simulink model "RaviDFG"  (R2023a)
settings: Solver=ode5  StartTime=0.0  StopTime=15  FixedStep=50e-9  MaxStep=1e-2  MinStep=1e-3  RelTol=1e-3  AbsTol=1e-3
undefined symbols (not defined in the file): d_base, d_Beta, d_bl, d_Cdc, d_Cf, d_ctg, d_GSC_IL1_iv, d_GSC_IL1_ki, d_GSC_IL1_kp, d_GSC_IL2_iv, d_GSC_IL2_ki, d_GSC_IL2_kp, d_GSC_OL1_iv, d_GSC_OL1_ki, d_GSC_OL1_kp, d_GSC_OL2_iv, d_GSC_OL2_ki, d_GSC_OL2_kp, d_Hg, d_Ht, d_igd, d_igq, d_iid, d_iiq, d_isd, d_isq, d_Kmrr, d_kopt, d_ktg, d_Lg, d_Li, d_Lm, d_Ls_d, d_MSC_IL1_iv, d_MSC_IL1_ki, d_MSC_IL1_kp, d_MSC_IL2_iv, d_MSC_IL2_ki, d_MSC_IL2_kp, d_MSC_OL1_iv, d_MSC_OL1_ki, d_MSC_OL1_kp, d_MSC_OL2_iv, d_MSC_OL2_ki, d_MSC_OL2_kp, d_Qs, d_R1, d_R2, d_Rc, d_Rg, d_Ri, d_Tr, d_Ts, d_vcd, d_vcq, d_VDC, d_vw, d_welb, d_wg, d_ws ... (+7)
libraries: eeGeneralControl x2, rtlab x2
settings Model: Creator=rpat227  LastModifiedBy=rufar
settings SolverCC: AlgebraicLoopSolver=TrustRegion
settings DebuggingCC: UnconnectedInputMsg=warning  UnconnectedOutputMsg=warning  UnconnectedLineMsg=warning
settings ModelReferenceCC: EnableRefExpFcnMdlSchedulingChecks=on

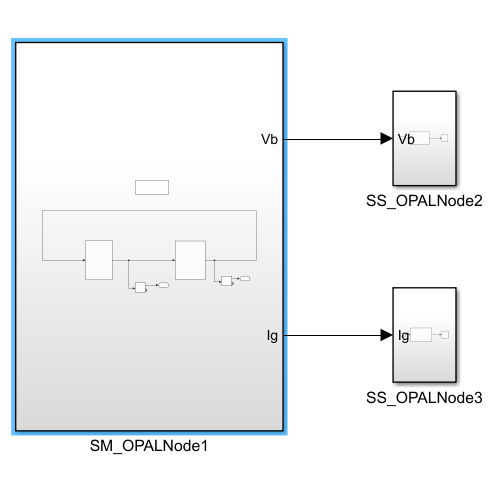
[thumbnail: Simulink's stored preview of the top-level diagram]
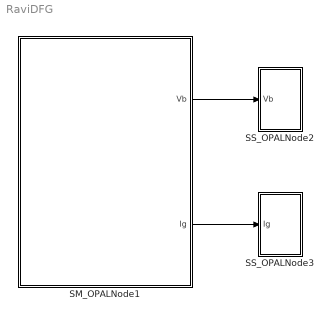
== system RaviDFG ==
  SM_OPALNode1 : Subsystem
  SS_OPALNode2 : Subsystem
  SS_OPALNode3 : Subsystem
  wires:
  SM_OPALNode1/1(Vb) -> SS_OPALNode2/1(Vb)
  SM_OPALNode1/2(Ig) -> SS_OPALNode3/1(Ig)

== system RaviDFG/SM_OPALNode1 ==
  Complex to Real-Imag : ComplexToRealImag
  Complex to Real-Imag1 : ComplexToRealImag
  DFIG : Subsystem
  Measurement : Subsystem
  Network : Subsystem
  Vb : Outport
  Ig : Outport  Port=2
  wires:
  DFIG/1(Ig) -> Complex to Real-Imag/1, Network/1(Ig)
  Network/1(Vb) -> Complex to Real-Imag1/1, DFIG/1(Vb)
  Complex to Real-Imag/1 -> Ig/1
  Complex to Real-Imag1/1 -> Vb/1

== system RaviDFG/SS_OPALNode2 ==
  Vb : Inport
  OpComm1 : rtlab/OpComm  nbport=1  groupe_acq=1  subsys_rate=0  st=0  Synchronization=on  Interpolation=on  Threshold=1.0  Missed_Data=off  Sim_Time=off  Samples=off  dynSigOut=off  from_console=0  warning_done=off  writeOpCommFile=off  Offset=off
      settings: SourceProductName=RT-LAB
  Vb_Scope : Scope
  wires:
  OpComm1/1 -> Vb_Scope/1
  Vb/1 -> OpComm1/1

== system RaviDFG/SS_OPALNode3 ==
  Ig : Inport
  Ig_Scope : Scope
  OpComm : rtlab/OpComm  nbport=1  groupe_acq=1  subsys_rate=0  st=0  Synchronization=on  Interpolation=on  Threshold=1.0  Missed_Data=off  Sim_Time=off  Samples=off  dynSigOut=off  from_console=0  warning_done=off  writeOpCommFile=off  Offset=off
      settings: SourceProductName=RT-LAB
  wires:
  OpComm/1 -> Ig_Scope/1
  Ig/1 -> OpComm/1

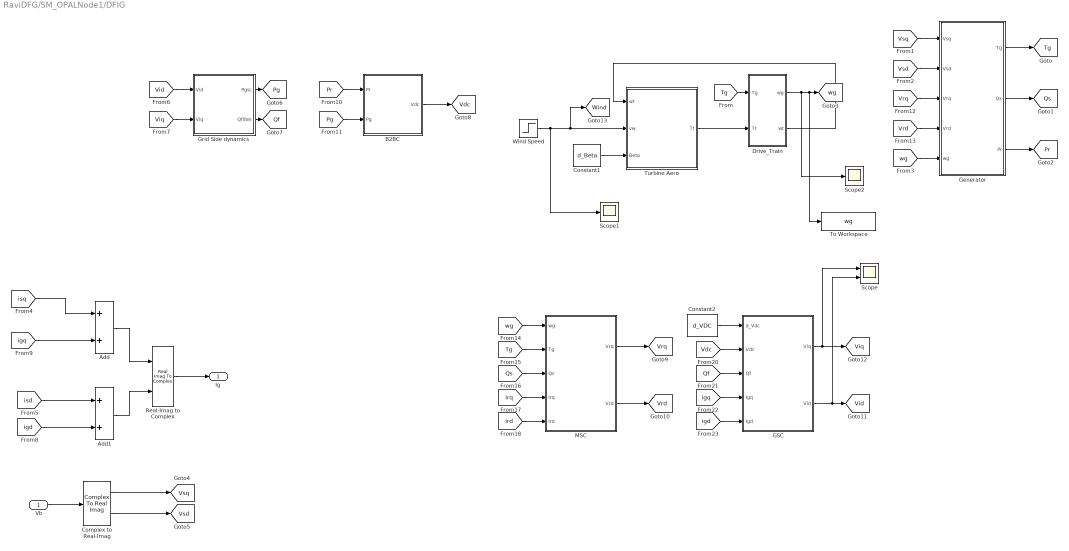
== system RaviDFG/SM_OPALNode1/DFIG ==
  Vb : Inport
  Add : Sum
  Add1 : Sum
  B2BC : Subsystem
  Complex to Real-Imag : ComplexToRealImag
  Constant1 : Constant  Value=d_Beta
  Constant2 : Constant  Value=d_VDC
  Drive_Train : Subsystem
  GSC : Subsystem
  Generator : Subsystem
  Grid Side dynamics : Subsystem
  MSC : Subsystem
  Real-Imag to Complex : RealImagToComplex
  Scope : Scope  NumInputPorts=2
  Scope1 : Scope
  Scope2 : Scope
  To Workspace : ToWorkspace  VariableName=wg  SaveFormat=Structure With Time  SampleTime=-1
  Turbine Aero : Subsystem
  Wind Speed : Step  Time=5  Before=d_vw  After=d_vw  SampleTime=0
  Ig : Outport
  tag scope: Pg=global, Pr=global, Qf=global, Qs=global, Tg=global, Vdc=global, Vid=global, Viq=global, Vrd=global, Vrq=global, Vsd=global, Vsq=global, Wind=global, wg=global
  wires:
  MSC/1(Vrq) -> [Vrq]
  [Pg] -> B2BC/2(Pg)
  [Viq] -> Grid Side dynamics/2(Viq)
  B2BC/1(Vdc) -> [Vdc]
  [Pr] -> B2BC/1(Pr)
  GSC/1(Viq) -> Scope/1, [Viq]
  Turbine Aero/1(Tt) -> Drive_Train/2(Tt)
  [irq] -> MSC/4(Irq)
  Wind Speed/1 -> Scope1/1, Turbine Aero/2(vw), [Wind]
  [Qs] -> MSC/3(Qs)
  [wg] -> MSC/1("wg ")
  Generator/3(Pr) -> [Pr]
  Drive_Train/1(wg) -> Scope2/1, To Workspace/1, [wg]
  [Qf] -> GSC/3(Qf)
  [Tg] -> MSC/2(Tg)
  Constant1/1 -> Turbine Aero/3(Beta)
  Grid Side dynamics/2(Qfilter) -> [Qf]
  [Tg] -> Drive_Train/1(Tg)
  [Vrq] -> Generator/3(Vrq)
  [Vrd] -> Generator/4(Vrd)
  [Vdc] -> GSC/2(Vdc)
  [igd] -> GSC/5(Igd)
  [Vid] -> Grid Side dynamics/1(Vid)
  Generator/2(Qs) -> [Qs]
  Generator/1(Tg) -> [Tg]
  [Vsd] -> Generator/2(Vsd)
  Grid Side dynamics/1(Pgsc) -> [Pg]
  [Vsq] -> Generator/1(Vsq)
  Drive_Train/2(wt) -> Turbine Aero/1(wt)
  [igq] -> GSC/4(Igq)
  MSC/2(Vrd) -> [Vrd]
  Constant2/1 -> GSC/1("d_Vdc ")
  GSC/2(Vid) -> Scope/2, [Vid]
  [wg] -> Generator/5(wg)
  [ird] -> MSC/5(Ird)
  [igd] -> Add1/2
  Add1/1 -> Real-Imag to Complex/2
  [igq] -> Add/2
  Add/1 -> Real-Imag to Complex/1
  [isd] -> Add1/1
  [isq] -> Add/1
  Real-Imag to Complex/1 -> Ig/1
  Vb/1 -> Complex to Real-Imag/1
  Complex to Real-Imag/2 -> [Vsd]
  Complex to Real-Imag/1 -> [Vsq]

== system RaviDFG/SM_OPALNode1/Measurement ==
  Scope{,1..7} (8 alike) : Scope
  To Workspace : ToWorkspace  VariableName=P  SaveFormat=Structure With Time  SampleTime=-1
  wires:
  [P] -> To Workspace/1, Scope/1
  [Vinf] -> Scope7/1
  [Bus] -> Scope6/1
  [Wind] -> Scope5/1
  [Vdc] -> Scope4/1
  [Qs] -> Scope3/1
  [Pr] -> Scope2/1
  [Ps] -> Scope1/1

== system RaviDFG/SM_OPALNode1/Network ==
  Ig : Inport
  Add2 : Sum
  Complex to Magnitude-Angle : ComplexToMagnitudeAngle
  Constant : Constant  Value=vinf
  Display : Display
  Display1 : Display
  Display2 : Display
  Gain : Gain  Gain=Znet
  Vb : Outport
  tag scope: Bus=global, Theta=global, Vinf=global
  wires:
  Gain/1 -> Add2/1
  Add2/1 -> Display1/1, Vb/1, Complex to Magnitude-Angle/1
  Complex to Magnitude-Angle/2 -> [Theta]
  Complex to Magnitude-Angle/1 -> Display2/1, [Bus]
  Ig/1 -> Display/1, Gain/1
  Constant/1 -> Add2/2, [Vinf]

== system RaviDFG/SM_OPALNode1/DFIG/B2BC ==
  Pr : Inport
  Pg : Inport  Port=2
  Add : Sum  Inputs=+-
  Divide : Product  Inputs=*/
  Gain : Gain  Gain=d_Cdc
  Integrator : Integrator  InitialCondition=d_VDC
  Scope : Scope
  Vdc : Outport
  wires:
  Pr/1 -> Add/1
  Pg/1 -> Add/2
  Add/1 -> Gain/1
  Gain/1 -> Divide/1
  Divide/1 -> Integrator/1
  Integrator/1 -> Divide/2, Scope/1, Vdc/1

== system RaviDFG/SM_OPALNode1/DFIG/Drive_Train ==
  Tg : Inport
  Tt : Inport  Port=2
  Add : Sum  Inputs=-+
  Add1 : Sum  Inputs=+-
  Add2 : Sum  Inputs=-+
  Add3 : Sum
  Gain : Gain  Gain=1./(2*d_Hg)
  Gain1 : Gain  Gain=1./(2*d_Ht)
  Gain2 : Gain  Gain=d_welb
  Gain3 : Gain  Gain=d_ktg
  Gain4 : Gain  Gain=d_ctg
  d_Ts : Integrator  InitialCondition=d_Ts
  d_wg : Integrator  InitialCondition=d_wg
  d_wt : Integrator  InitialCondition=d_wt
  wg : Outport
  wt : Outport  Port=2
  wires:
  Tg/1 -> Add/1
  Tt/1 -> Add1/1
  Add/1 -> Gain/1
  Add1/1 -> Gain1/1
  Gain/1 -> d_wg/1
  Gain1/1 -> d_wt/1
  d_wg/1 -> wg/1, Add2/1
  d_wt/1 -> Add2/2, wt/1
  Add2/1 -> Gain2/1
  Gain2/1 -> Gain4/1, Gain3/1
  Gain3/1 -> d_Ts/1
  d_Ts/1 -> Add3/1
  Gain4/1 -> Add3/2
  Add3/1 -> Add/2, Add1/2

== system RaviDFG/SM_OPALNode1/DFIG/GSC ==
  "d_Vdc " : Inport
  Vdc : Inport  Port=2
  Qf : Inport  Port=3
  Igq : Inport  Port=4
  Igd : Inport  Port=5
  Add{,1..3} (4 alike) : Sum  Inputs=+-
  Constant : Constant  Value=0
  GSC_IL_1 : Subsystem
  GSC_IL_2 : Subsystem
  GSC_OL_1 : Subsystem
  GSC_OL_2 : Subsystem
  Subsystem : Subsystem
  Subsystem1 : Subsystem
  Viq : Outport
  Vid : Outport  Port=2
  wires:
  "d_Vdc "/1 -> Add/1
  Vdc/1 -> Add/2
  Add/1 -> GSC_OL_1/1(In1)
  GSC_OL_1/1(Out1) -> Add1/1
  Add1/1 -> GSC_IL_1/1(In1)
  Add2/1 -> GSC_OL_2/1(In1)
  GSC_OL_2/1(Out1) -> Add3/1
  Add3/1 -> GSC_IL_2/1(In1)
  Constant/1 -> Add2/1
  Qf/1 -> Add2/2
  Subsystem/1(Igq') -> Add1/2
  Subsystem/2(Igd') -> Add3/2
  Igq/1 -> Subsystem/1(Igq)
  Igd/1 -> Subsystem/2(Igd)
  GSC_IL_1/1(Out1) -> Subsystem1/1(Viq')
  GSC_IL_2/1(Out1) -> Subsystem1/2(Vid')
  Subsystem1/1(Viq) -> Viq/1
  Subsystem1/2(Vid) -> Vid/1

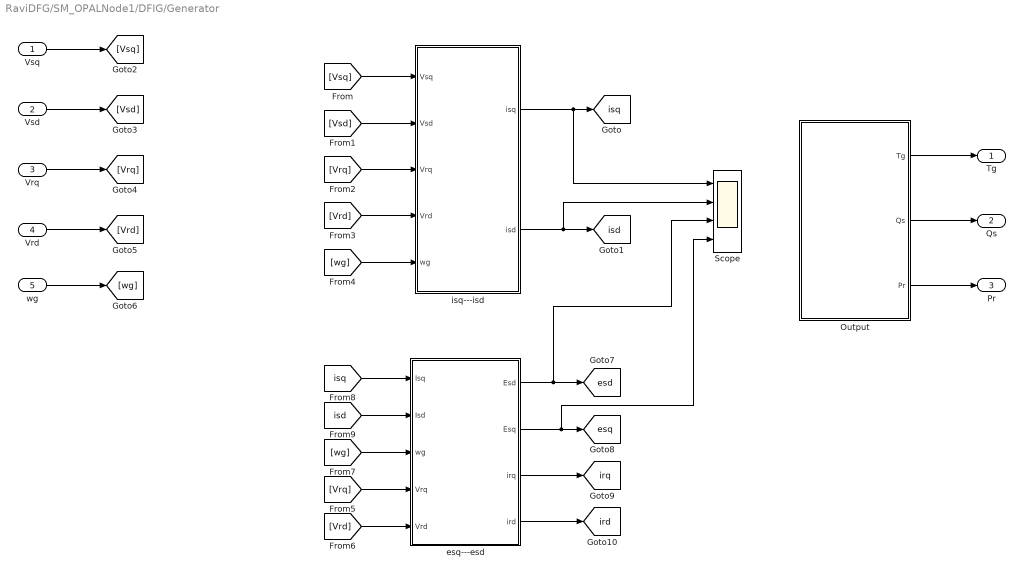
== system RaviDFG/SM_OPALNode1/DFIG/Generator ==
  Vsq : Inport
  Vsd : Inport  Port=2
  Vrq : Inport  Port=3
  Vrd : Inport  Port=4
  wg : Inport  Port=5
  Output : Subsystem
  Scope : Scope  NumInputPorts=4
  esq---esd : Subsystem
  isq---isd : Subsystem
  Tg : Outport
  Qs : Outport  Port=2
  Pr : Outport  Port=3
  tag scope: esd=global, esq=global, ird=global, irq=global, isd=global, isq=global
  wires:
  [Vsq] -> isq---isd/1(Vsq)
  [Vsd] -> isq---isd/2(Vsd)
  [Vrq] -> isq---isd/3(Vrq)
  [Vrd] -> isq---isd/4(Vrd)
  [wg] -> isq---isd/5(wg)
  isq---isd/1(isq) -> Scope/1, [isq]
  isq---isd/2(isd) -> Scope/2, [isd]
  Vsq/1 -> [Vsq]
  Vsd/1 -> [Vsd]
  Vrq/1 -> [Vrq]
  Vrd/1 -> [Vrd]
  wg/1 -> [wg]
  [Vrq] -> esq---esd/4(Vrq)
  [Vrd] -> esq---esd/5(Vrd)
  [wg] -> esq---esd/3(wg)
  [isq] -> esq---esd/1(Isq)
  [isd] -> esq---esd/2(Isd)
  esq---esd/2(Esq) -> Scope/4, [esq]
  esq---esd/3(irq) -> [irq]
  esq---esd/4(ird) -> [ird]
  Output/1(Tg) -> Tg/1
  Output/2(Qs) -> Qs/1
  Output/3(Pr) -> Pr/1
  esq---esd/1(Esd) -> Scope/3, [esd]

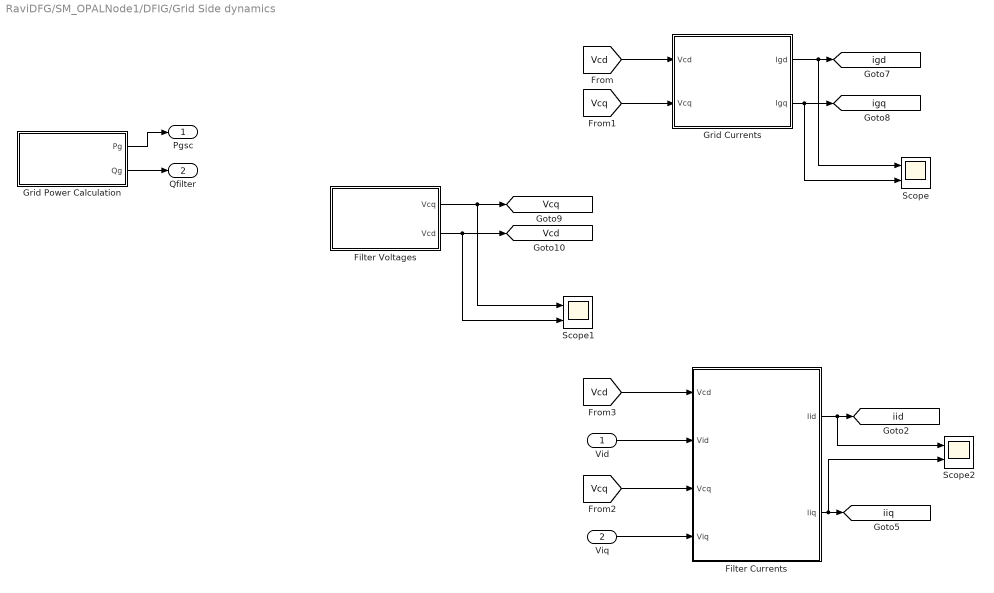
== system RaviDFG/SM_OPALNode1/DFIG/Grid Side dynamics ==
  Vid : Inport
  Viq : Inport  Port=2
  Filter Currents : Subsystem
  Filter Voltages : Subsystem
  Grid Currents : Subsystem
  Grid Power Calculation : Subsystem
  Scope : Scope  NumInputPorts=2
  Scope1 : Scope  NumInputPorts=2
  Scope2 : Scope  NumInputPorts=2
  Pgsc : Outport
  Qfilter : Outport  Port=2
  tag scope: Vcd=global, Vcq=global, igd=global, igq=global, iid=global, iiq=global
  wires:
  Grid Currents/1(Igd) -> Scope/1, [igd]
  Filter Voltages/2(Vcd) -> Scope1/2, [Vcd]
  Viq/1 -> Filter Currents/4(Viq)
  Vid/1 -> Filter Currents/2(Vid)
  [Vcd] -> Filter Currents/1(Vcd)
  [Vcq] -> Filter Currents/3(Vcq)
  Filter Voltages/1(Vcq) -> Scope1/1, [Vcq]
  [Vcq] -> Grid Currents/2(Vcq)
  Filter Currents/1(Iid) -> Scope2/1, [iid]
  Filter Currents/2(Iiq) -> Scope2/2, [iiq]
  [Vcd] -> Grid Currents/1(Vcd)
  Grid Power Calculation/1(Pg) -> Pgsc/1
  Grid Power Calculation/2(Qg) -> Qfilter/1
  Grid Currents/2(Igq) -> Scope/2, [igq]

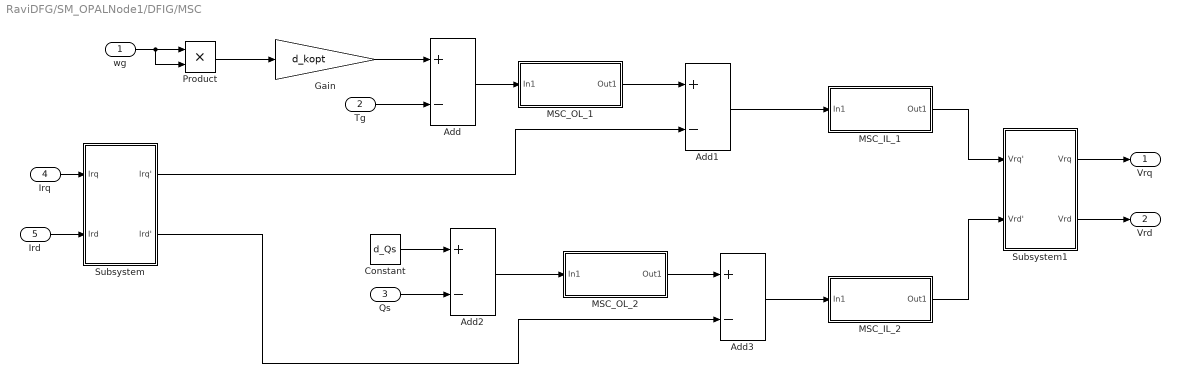
== system RaviDFG/SM_OPALNode1/DFIG/MSC ==
  "wg " : Inport
  Tg : Inport  Port=2
  Qs : Inport  Port=3
  Irq : Inport  Port=4
  Ird : Inport  Port=5
  Add{,1..3} (4 alike) : Sum  Inputs=+-
  Constant : Constant  Value=d_Qs
  Gain : Gain  Gain=d_kopt
  MSC_IL_1 : Subsystem
  MSC_IL_2 : Subsystem
  MSC_OL_1 : Subsystem
  MSC_OL_2 : Subsystem
  Product : Product
  Subsystem : Subsystem
  Subsystem1 : Subsystem
  Vrq : Outport
  Vrd : Outport  Port=2
  wires:
  "wg "/1 -> Product/2, Product/1
  Product/1 -> Gain/1
  Gain/1 -> Add/1
  Tg/1 -> Add/2
  Add/1 -> MSC_OL_1/1(In1)
  MSC_OL_1/1(Out1) -> Add1/1
  Add1/1 -> MSC_IL_1/1(In1)
  Add2/1 -> MSC_OL_2/1(In1)
  MSC_OL_2/1(Out1) -> Add3/1
  Add3/1 -> MSC_IL_2/1(In1)
  Constant/1 -> Add2/1
  Qs/1 -> Add2/2
  Subsystem/1(Irq') -> Add1/2
  Subsystem/2(Ird') -> Add3/2
  Irq/1 -> Subsystem/1(Irq)
  Ird/1 -> Subsystem/2(Ird)
  MSC_IL_1/1(Out1) -> Subsystem1/1(Vrq')
  MSC_IL_2/1(Out1) -> Subsystem1/2(Vrd')
  Subsystem1/1(Vrq) -> Vrq/1
  Subsystem1/2(Vrd) -> Vrd/1

== system RaviDFG/SM_OPALNode1/DFIG/Turbine Aero ==
  wt : Inport
  vw : Inport  Port=2
  Beta : Inport  Port=3
  Constant : Constant  Value=0.5*rho*pi*d_bl^2
  Constant4 : Constant  Value=3
  "Cp Calculation " : Subsystem
  Divide : Product  Inputs=*/
  Divide1 : Product  Inputs=*/
  Gain : Gain  Gain=d_wtrated*d_bl
  Gain1 : Gain  Gain=1/(d_base*10^6)
  Power : Math  Operator=pow
  Product : Product  Inputs=3
  Tt : Outport
  wires:
  Divide/1 -> "Cp Calculation "/1(Lambda)
  Product/1 -> Gain1/1
  Gain/1 -> Divide/1
  Power/1 -> Product/3
  vw/1 -> Power/1, Divide/2
  Constant4/1 -> Power/2
  "Cp Calculation "/1(Cp) -> Product/2
  Divide1/1 -> Tt/1
  wt/1 -> Divide1/2, Gain/1
  Beta/1 -> "Cp Calculation "/2(Beta)
  Gain1/1 -> Divide1/1
  Constant/1 -> Product/1

== system RaviDFG/SM_OPALNode1/DFIG/GSC/GSC_IL_1 ==
  In1 : Inport
  Gain : Gain  Gain=d_GSC_IL1_ki
  Gain1 : Gain  Gain=d_GSC_IL1_kp
  Integrator : Integrator  InitialCondition=d_GSC_IL1_iv
  Sum : Sum  Inputs=|++
  Out1 : Outport
  wires:
  Gain/1 -> Integrator/1
  Integrator/1 -> Sum/1
  Gain1/1 -> Sum/2
  Sum/1 -> Out1/1
  In1/1 -> Gain1/1, Gain/1

== system RaviDFG/SM_OPALNode1/DFIG/GSC/GSC_IL_2 ==
  In1 : Inport
  Gain : Gain  Gain=d_GSC_IL2_ki
  Gain1 : Gain  Gain=d_GSC_IL2_kp
  Integrator : Integrator  InitialCondition=d_GSC_IL2_iv
  Sum : Sum  Inputs=|++
  Out1 : Outport
  wires:
  Gain/1 -> Integrator/1
  Integrator/1 -> Sum/1
  Gain1/1 -> Sum/2
  Sum/1 -> Out1/1
  In1/1 -> Gain1/1, Gain/1

== system RaviDFG/SM_OPALNode1/DFIG/GSC/GSC_OL_1 ==
  In1 : Inport
  Gain : Gain  Gain=d_GSC_OL1_ki
  Gain1 : Gain  Gain=d_GSC_OL1_kp
  Integrator : Integrator  InitialCondition=d_GSC_OL1_iv
  Sum : Sum  Inputs=|++
  Out1 : Outport
  wires:
  Gain/1 -> Integrator/1
  Integrator/1 -> Sum/1
  Gain1/1 -> Sum/2
  Sum/1 -> Out1/1
  In1/1 -> Gain1/1, Gain/1

== system RaviDFG/SM_OPALNode1/DFIG/GSC/GSC_OL_2 ==
  In1 : Inport
  Gain : Gain  Gain=d_GSC_OL2_ki
  Gain1 : Gain  Gain=d_GSC_OL2_kp
  Integrator : Integrator  InitialCondition=d_GSC_OL2_iv
  Sum : Sum  Inputs=|++
  Out1 : Outport
  wires:
  Gain/1 -> Integrator/1
  Integrator/1 -> Sum/1
  Gain1/1 -> Sum/2
  Sum/1 -> Out1/1
  In1/1 -> Gain1/1, Gain/1

== system RaviDFG/SM_OPALNode1/DFIG/GSC/Subsystem ==
  Igq : Inport
  Igd : Inport  Port=2
  Complex to Real-Imag : ComplexToRealImag
  Gain : Gain  Gain=-j
  Math Function : Math
  Product : Product
  Real-Imag to Complex : RealImagToComplex
  Igq' : Outport
  Igd' : Outport  Port=2
  wires:
  Igd/1 -> Real-Imag to Complex/2
  Real-Imag to Complex/1 -> Product/1
  Gain/1 -> Math Function/1
  Complex to Real-Imag/2 -> Igd'/1
  Product/1 -> Complex to Real-Imag/1
  [Theta] -> Gain/1
  Complex to Real-Imag/1 -> Igq'/1
  Math Function/1 -> Product/2
  Igq/1 -> Real-Imag to Complex/1

== system RaviDFG/SM_OPALNode1/DFIG/GSC/Subsystem1 ==
  Viq' : Inport
  Vid' : Inport  Port=2
  Complex to Real-Imag : ComplexToRealImag
  Gain : Gain  Gain=j
  Math Function : Math
  Product : Product
  Real-Imag to Complex : RealImagToComplex
  Viq : Outport
  Vid : Outport  Port=2
  wires:
  Vid'/1 -> Real-Imag to Complex/2
  Real-Imag to Complex/1 -> Product/1
  Gain/1 -> Math Function/1
  Complex to Real-Imag/2 -> Vid/1
  Product/1 -> Complex to Real-Imag/1
  [Theta] -> Gain/1
  Complex to Real-Imag/1 -> Viq/1
  Math Function/1 -> Product/2
  Viq'/1 -> Real-Imag to Complex/1

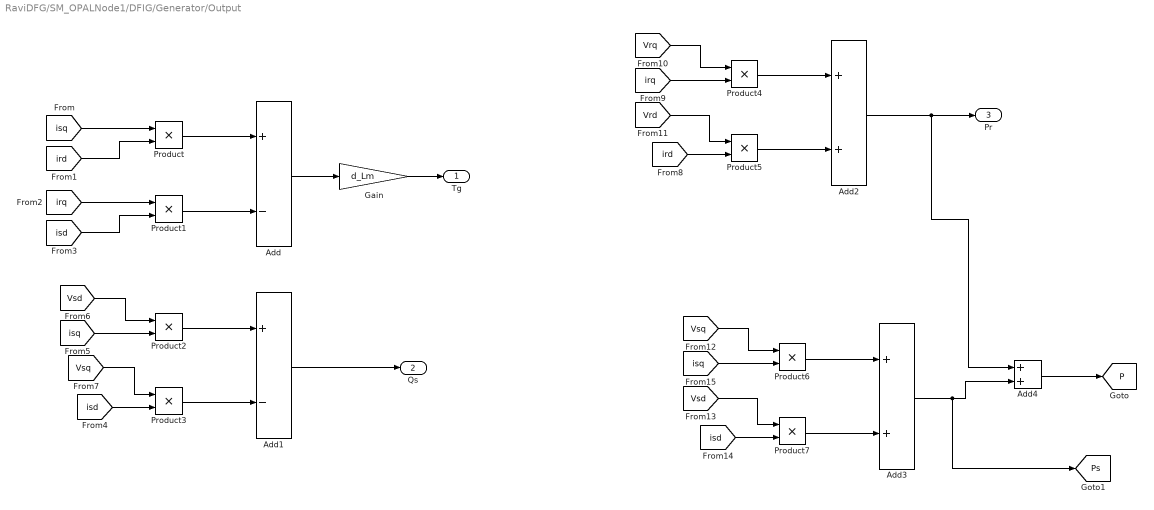
== system RaviDFG/SM_OPALNode1/DFIG/Generator/Output ==
  Add : Sum  Inputs=+-
  Add1 : Sum  Inputs=+-
  Add2 : Sum
  Add3 : Sum
  Add4 : Sum
  Gain : Gain  Gain=d_Lm
  Product{,1..7} (8 alike) : Product
  Tg : Outport
  Qs : Outport  Port=2
  Pr : Outport  Port=3
  tag scope: P=global, Ps=global
  wires:
  Add/1 -> Gain/1
  Product/1 -> Add/1
  Product1/1 -> Add/2
  [isq] -> Product/1
  [ird] -> Product/2
  [irq] -> Product1/1
  [isd] -> Product1/2
  Gain/1 -> Tg/1
  Product2/1 -> Add1/1
  Product3/1 -> Add1/2
  [isd] -> Product3/2
  [isq] -> Product2/2
  [Vsd] -> Product2/1
  [Vsq] -> Product3/1
  Add1/1 -> Qs/1
  [ird] -> Product5/2
  Product4/1 -> Add2/1
  Product5/1 -> Add2/2
  Add2/1 -> Add4/1, Pr/1
  [irq] -> Product4/2
  [Vrq] -> Product4/1
  [Vrd] -> Product5/1
  [isd] -> Product7/2
  Product6/1 -> Add3/1
  [isq] -> Product6/2
  [Vsq] -> Product6/1
  Product7/1 -> Add3/2
  [Vsd] -> Product7/1
  Add3/1 -> [Ps], Add4/2
  Add4/1 -> [P]

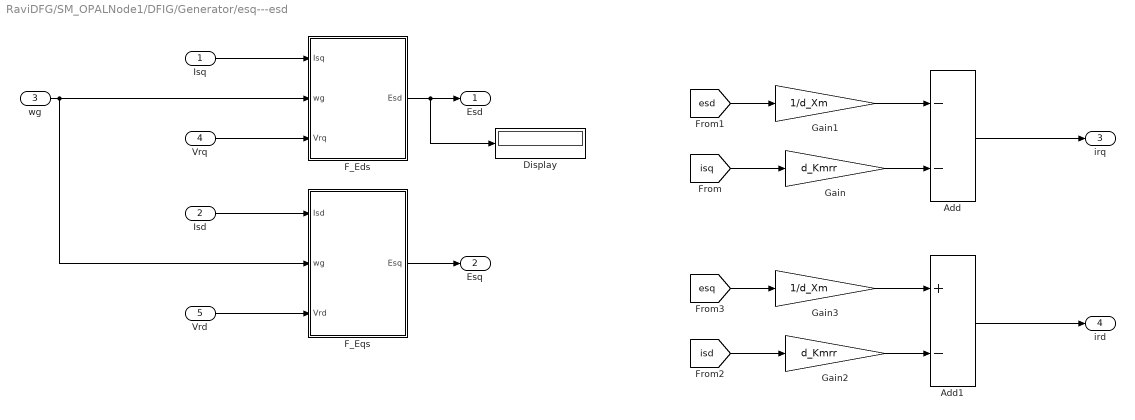
== system RaviDFG/SM_OPALNode1/DFIG/Generator/esq---esd ==
  Isq : Inport
  Isd : Inport  Port=2
  wg : Inport  Port=3
  Vrq : Inport  Port=4
  Vrd : Inport  Port=5
  Add : Sum  Inputs=--
  Add1 : Sum  Inputs=+-
  Display : Display
  F_Eds : Subsystem
  F_Eqs : Subsystem
  Gain : Gain  Gain=d_Kmrr
  Gain1 : Gain  Gain=1/d_Xm
  Gain2 : Gain  Gain=d_Kmrr
  Gain3 : Gain  Gain=1/d_Xm
  Esd : Outport
  Esq : Outport  Port=2
  irq : Outport  Port=3
  ird : Outport  Port=4
  wires:
  F_Eds/1(Esd) -> Display/1, Esd/1
  F_Eqs/1(Esq) -> Esq/1
  Isq/1 -> F_Eds/1(Isq)
  Isd/1 -> F_Eqs/1(Isd)
  wg/1 -> F_Eqs/2(wg), F_Eds/2(wg)
  Vrq/1 -> F_Eds/3(Vrq)
  Vrd/1 -> F_Eqs/3(Vrd)
  Gain/1 -> Add/2
  [isq] -> Gain/1
  Gain1/1 -> Add/1
  [esd] -> Gain1/1
  Add/1 -> irq/1
  [isd] -> Gain2/1
  Gain2/1 -> Add1/2
  [esq] -> Gain3/1
  Add1/1 -> ird/1
  Gain3/1 -> Add1/1

== system RaviDFG/SM_OPALNode1/DFIG/Generator/isq---isd ==
  Vsq : Inport
  Vsd : Inport  Port=2
  Vrq : Inport  Port=3
  Vrd : Inport  Port=4
  wg : Inport  Port=5
  Display : Display
  Display1 : Display
  F_Ids : Subsystem
  F_Iqs : Subsystem
  isq : Outport
  isd : Outport  Port=2
  wires:
  F_Iqs/1(Isq) -> Display/1, isq/1
  Vsq/1 -> F_Iqs/1(Vsq)
  Vsd/1 -> F_Ids/1(Vsd)
  Vrq/1 -> F_Iqs/2(Vrq)
  Vrd/1 -> F_Ids/2(Vrd)
  wg/1 -> F_Iqs/3(wg), F_Ids/3(wg)
  F_Ids/1(Isd) -> Display1/1, isd/1

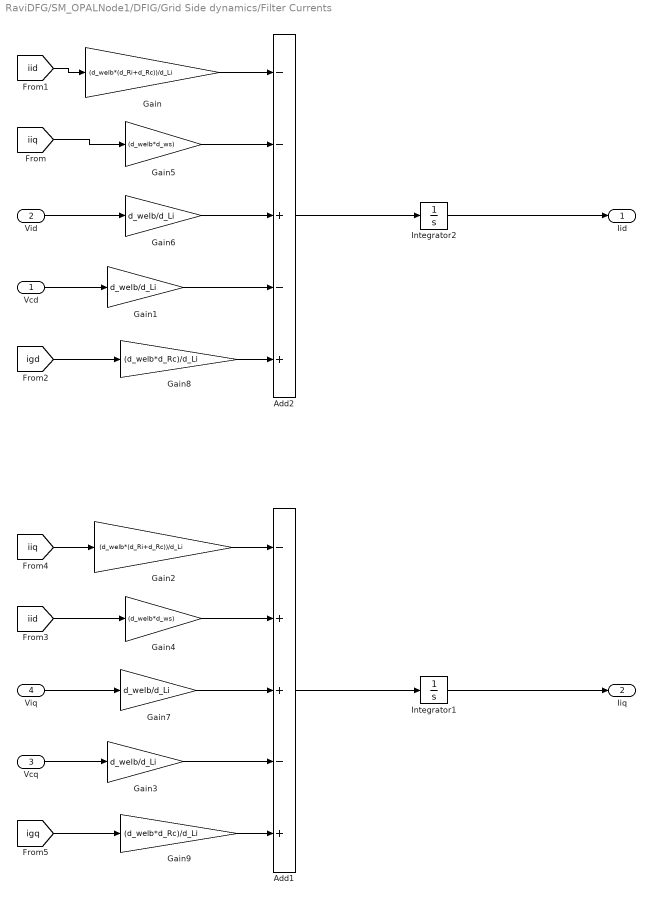
== system RaviDFG/SM_OPALNode1/DFIG/Grid Side dynamics/Filter Currents ==
  Vcd : Inport
  Vid : Inport  Port=2
  Vcq : Inport  Port=3
  Viq : Inport  Port=4
  Add1 : Sum  Inputs=-++-+
  Add2 : Sum  Inputs=--+-+
  Gain : Gain  Gain=(d_welb*(d_Ri+d_Rc))/d_Li
  Gain{1,3,6..7} (4 alike) : Gain  Gain=d_welb/d_Li
  Gain2 : Gain  Gain=(d_welb*(d_Ri+d_Rc))/d_Li
  Gain4 : Gain  Gain=(d_welb*d_ws)
  Gain5 : Gain  Gain=(d_welb*d_ws)
  Gain8 : Gain  Gain=(d_welb*d_Rc)/d_Li
  Gain9 : Gain  Gain=(d_welb*d_Rc)/d_Li
  Integrator1 : Integrator  InitialCondition=d_iiq  UpperSaturationLimit=1  LowerSaturationLimit=-1
  Integrator2 : Integrator  InitialCondition=d_iid  UpperSaturationLimit=1  LowerSaturationLimit=-1
  Iid : Outport
  Iiq : Outport  Port=2
  wires:
  Gain5/1 -> Add2/2
  Gain6/1 -> Add2/3
  [iiq] -> Gain5/1
  Vid/1 -> Gain6/1
  Add2/1 -> Integrator2/1
  Gain/1 -> Add2/1
  [iid] -> Gain/1
  Gain1/1 -> Add2/4
  Vcd/1 -> Gain1/1
  Integrator2/1 -> Iid/1
  Gain8/1 -> Add2/5
  [igd] -> Gain8/1
  Add1/1 -> Integrator1/1
  Integrator1/1 -> Iiq/1
  Gain7/1 -> Add1/3
  Gain3/1 -> Add1/4
  [iiq] -> Gain2/1
  Gain2/1 -> Add1/1
  Viq/1 -> Gain7/1
  [igq] -> Gain9/1
  Vcq/1 -> Gain3/1
  [iid] -> Gain4/1
  Gain4/1 -> Add1/2
  Gain9/1 -> Add1/5

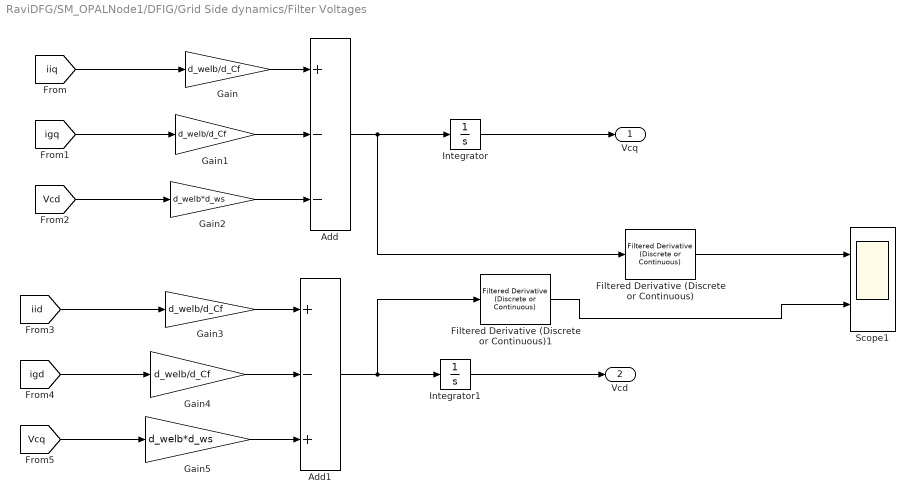
== system RaviDFG/SM_OPALNode1/DFIG/Grid Side dynamics/Filter Voltages ==
  Add : Sum  Inputs=+--
  Add1 : Sum  Inputs=+-+
  Filtered Derivative (Discrete or Continuous) : eeGeneralControl/Filtered Derivative (Discrete or Continuous)  K=1  T=0.9  B=inf  A=-inf  minRatio=10  init_option=Inherited from block input  x0=0  Ts=0
  Filtered Derivative (Discrete or Continuous)1 : eeGeneralControl/Filtered Derivative (Discrete or Continuous)  K=1  T=0.9  B=inf  A=-inf  minRatio=10  init_option=Inherited from block input  x0=0  Ts=0
  Gain{,1,3..4} (4 alike) : Gain  Gain=d_welb/d_Cf
  Gain2 : Gain  Gain=d_welb*d_ws
  Gain5 : Gain  Gain=d_welb*d_ws
  Integrator : Integrator  InitialCondition=d_vcq
  Integrator1 : Integrator  InitialCondition=d_vcd
  Scope1 : Scope  NumInputPorts=2
  Vcq : Outport
  Vcd : Outport  Port=2
  wires:
  [iiq] -> Gain/1
  [igq] -> Gain1/1
  Gain/1 -> Add/1
  Gain1/1 -> Add/2
  Gain2/1 -> Add/3
  [Vcd] -> Gain2/1
  Integrator/1 -> Vcq/1
  Gain5/1 -> Add1/3
  Integrator1/1 -> Vcd/1
  [Vcq] -> Gain5/1
  Gain4/1 -> Add1/2
  Gain3/1 -> Add1/1
  [igd] -> Gain4/1
  [iid] -> Gain3/1
  Add1/1 -> Filtered Derivative (Discrete or Continuous)1/1, Integrator1/1
  Add/1 -> Filtered Derivative (Discrete or Continuous)/1, Integrator/1
  Filtered Derivative (Discrete or Continuous)/1 -> Scope1/1
  Filtered Derivative (Discrete or Continuous)1/1 -> Scope1/2

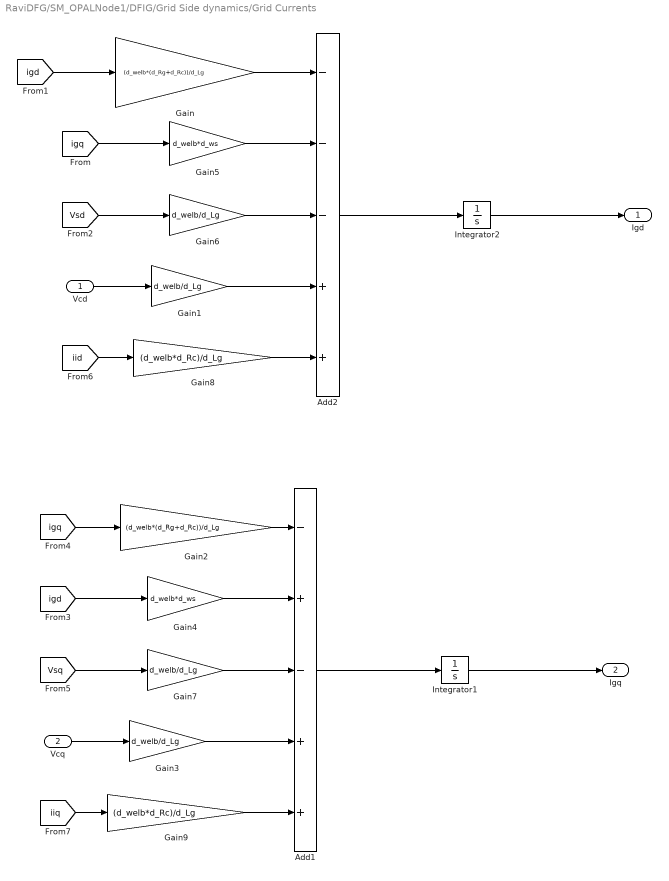
== system RaviDFG/SM_OPALNode1/DFIG/Grid Side dynamics/Grid Currents ==
  Vcd : Inport
  Vcq : Inport  Port=2
  Add1 : Sum  Inputs=-+-++
  Add2 : Sum  Inputs=---++
  Gain : Gain  Gain=(d_welb*(d_Rg+d_Rc))/d_Lg
  Gain{1,3,6..7} (4 alike) : Gain  Gain=d_welb/d_Lg
  Gain2 : Gain  Gain=(d_welb*(d_Rg+d_Rc))/d_Lg
  Gain4 : Gain  Gain=d_welb*d_ws
  Gain5 : Gain  Gain=d_welb*d_ws
  Gain8 : Gain  Gain=(d_welb*d_Rc)/d_Lg
  Gain9 : Gain  Gain=(d_welb*d_Rc)/d_Lg
  Integrator1 : Integrator  InitialCondition=d_igq  UpperSaturationLimit=1  LowerSaturationLimit=-1
  Integrator2 : Integrator  InitialCondition=d_igd  UpperSaturationLimit=1  LowerSaturationLimit=-1
  Igd : Outport
  Igq : Outport  Port=2
  wires:
  Gain5/1 -> Add2/2
  Gain6/1 -> Add2/3
  [igq] -> Gain5/1
  [Vsd] -> Gain6/1
  Add2/1 -> Integrator2/1
  Gain/1 -> Add2/1
  [igd] -> Gain/1
  Gain1/1 -> Add2/4
  Vcd/1 -> Gain1/1
  Integrator2/1 -> Igd/1
  Gain8/1 -> Add2/5
  [iid] -> Gain8/1
  [iiq] -> Gain9/1
  Gain9/1 -> Add1/5
  Integrator1/1 -> Igq/1
  [igq] -> Gain2/1
  [Vsq] -> Gain7/1
  Vcq/1 -> Gain3/1
  [igd] -> Gain4/1
  Gain3/1 -> Add1/4
  Gain7/1 -> Add1/3
  Add1/1 -> Integrator1/1
  Gain2/1 -> Add1/1
  Gain4/1 -> Add1/2

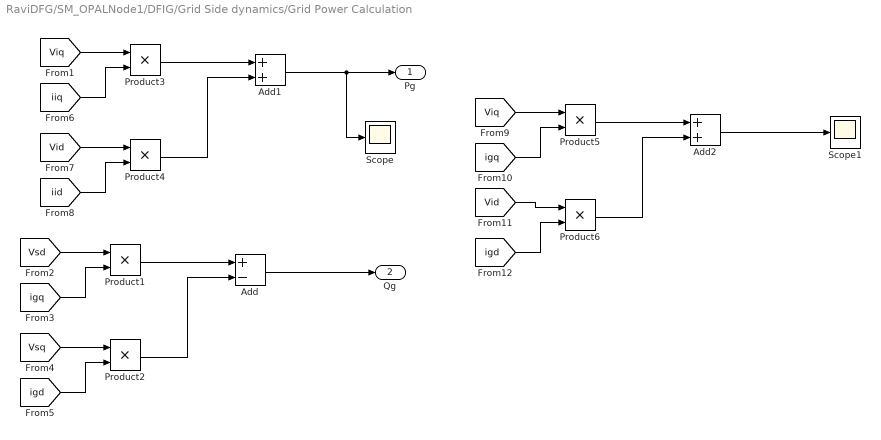
== system RaviDFG/SM_OPALNode1/DFIG/Grid Side dynamics/Grid Power Calculation ==
  Add : Sum  Inputs=+-
  Add1 : Sum
  Add2 : Sum
  Product{1..6} (6 alike) : Product
  Scope : Scope
  Scope1 : Scope
  Pg : Outport
  Qg : Outport  Port=2
  wires:
  [Vsd] -> Product1/1
  [igq] -> Product1/2
  Product1/1 -> Add/1
  Add/1 -> Qg/1
  [Vsq] -> Product2/1
  [igd] -> Product2/2
  Product2/1 -> Add/2
  Product4/1 -> Add1/2
  [iid] -> Product4/2
  Add1/1 -> Scope/1, Pg/1
  [Vid] -> Product4/1
  Product3/1 -> Add1/1
  [Viq] -> Product3/1
  [iiq] -> Product3/2
  Product5/1 -> Add2/1
  [Vid] -> Product6/1
  [Viq] -> Product5/1
  [igq] -> Product5/2
  Add2/1 -> Scope1/1
  [igd] -> Product6/2
  Product6/1 -> Add2/2

== system RaviDFG/SM_OPALNode1/DFIG/MSC/MSC_IL_1 ==
  In1 : Inport
  Gain : Gain  Gain=d_MSC_IL1_ki
  Gain1 : Gain  Gain=d_MSC_IL1_kp
  Integrator : Integrator  InitialCondition=d_MSC_IL1_iv
  Sum : Sum  Inputs=|++
  Out1 : Outport
  wires:
  Gain/1 -> Integrator/1
  Integrator/1 -> Sum/1
  Gain1/1 -> Sum/2
  Sum/1 -> Out1/1
  In1/1 -> Gain1/1, Gain/1

== system RaviDFG/SM_OPALNode1/DFIG/MSC/MSC_IL_2 ==
  In1 : Inport
  Gain : Gain  Gain=d_MSC_IL2_ki
  Gain1 : Gain  Gain=d_MSC_IL2_kp
  Integrator : Integrator  InitialCondition=d_MSC_IL2_iv
  Sum : Sum  Inputs=|++
  Out1 : Outport
  wires:
  Gain/1 -> Integrator/1
  Integrator/1 -> Sum/1
  Gain1/1 -> Sum/2
  Sum/1 -> Out1/1
  In1/1 -> Gain1/1, Gain/1

== system RaviDFG/SM_OPALNode1/DFIG/MSC/MSC_OL_1 ==
  In1 : Inport
  Gain : Gain  Gain=d_MSC_OL1_ki
  Gain1 : Gain  Gain=d_MSC_OL1_kp
  Integrator : Integrator  InitialCondition=d_MSC_OL1_iv
  Sum : Sum  Inputs=|++
  Out1 : Outport
  wires:
  Gain/1 -> Integrator/1
  Integrator/1 -> Sum/1
  Gain1/1 -> Sum/2
  Sum/1 -> Out1/1
  In1/1 -> Gain1/1, Gain/1

== system RaviDFG/SM_OPALNode1/DFIG/MSC/MSC_OL_2 ==
  In1 : Inport
  Gain : Gain  Gain=d_MSC_OL2_ki
  Gain1 : Gain  Gain=d_MSC_OL2_kp
  Integrator : Integrator  InitialCondition=d_MSC_OL2_iv
  Sum : Sum  Inputs=|++
  Out1 : Outport
  wires:
  Gain/1 -> Integrator/1
  Integrator/1 -> Sum/1
  Gain1/1 -> Sum/2
  Sum/1 -> Out1/1
  In1/1 -> Gain1/1, Gain/1

== system RaviDFG/SM_OPALNode1/DFIG/MSC/Subsystem ==
  Irq : Inport
  Ird : Inport  Port=2
  Complex to Real-Imag : ComplexToRealImag
  Gain : Gain  Gain=-j
  Math Function : Math
  Product : Product
  Real-Imag to Complex : RealImagToComplex
  Irq' : Outport
  Ird' : Outport  Port=2
  wires:
  Ird/1 -> Real-Imag to Complex/2
  Real-Imag to Complex/1 -> Product/1
  Gain/1 -> Math Function/1
  Complex to Real-Imag/2 -> Ird'/1
  Product/1 -> Complex to Real-Imag/1
  [Theta] -> Gain/1
  Complex to Real-Imag/1 -> Irq'/1
  Math Function/1 -> Product/2
  Irq/1 -> Real-Imag to Complex/1

== system RaviDFG/SM_OPALNode1/DFIG/MSC/Subsystem1 ==
  Vrq' : Inport
  Vrd' : Inport  Port=2
  Complex to Real-Imag : ComplexToRealImag
  Gain : Gain  Gain=j
  Math Function : Math
  Product : Product
  Real-Imag to Complex : RealImagToComplex
  Vrq : Outport
  Vrd : Outport  Port=2
  wires:
  Vrd'/1 -> Real-Imag to Complex/2
  Real-Imag to Complex/1 -> Product/1
  Gain/1 -> Math Function/1
  Complex to Real-Imag/2 -> Vrd/1
  Product/1 -> Complex to Real-Imag/1
  [Theta] -> Gain/1
  Complex to Real-Imag/1 -> Vrq/1
  Math Function/1 -> Product/2
  Vrq'/1 -> Real-Imag to Complex/1

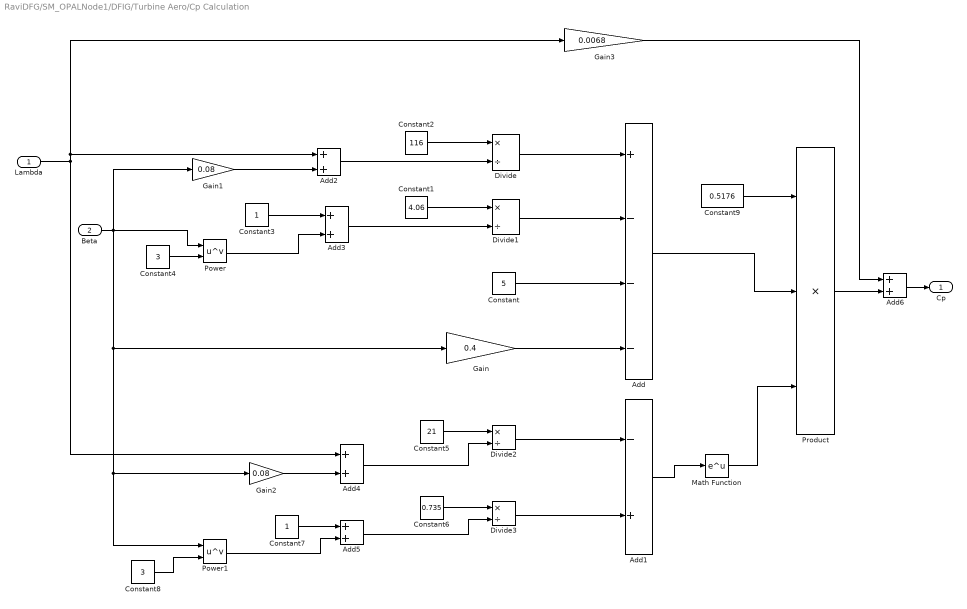
== system RaviDFG/SM_OPALNode1/DFIG/Turbine Aero/Cp Calculation  ==
  Lambda : Inport
  Beta : Inport  Port=2
  Add : Sum  Inputs=+---
  Add1 : Sum  Inputs=-+
  Add{2..6} (5 alike) : Sum
  Constant : Constant  Value=5
  Constant1 : Constant  Value=4.06
  Constant2 : Constant  Value=116
  Constant3 : Constant
  Constant4 : Constant  Value=3
  Constant5 : Constant  Value=21
  Constant6 : Constant  Value=0.735
  Constant7 : Constant
  Constant8 : Constant  Value=3
  Constant9 : Constant  Value=0.5176
  Divide{,1..3} (4 alike) : Product  Inputs=*/
  Gain : Gain  Gain=0.4
  Gain1 : Gain  Gain=0.08
  Gain2 : Gain  Gain=0.08
  Gain3 : Gain  Gain=0.0068
  Math Function : Math
  Power : Math  Operator=pow
  Power1 : Math  Operator=pow
  Product : Product  Inputs=3
  Cp : Outport
  wires:
  Power/1 -> Add3/2
  Add6/1 -> Cp/1
  Constant5/1 -> Divide2/1
  Constant6/1 -> Divide3/1
  Divide/1 -> Add/1
  Add3/1 -> Divide1/2
  Gain3/1 -> Add6/1
  Constant4/1 -> Power/2
  Constant/1 -> Add/3
  Beta/1 -> Gain1/1, Gain/1, Gain2/1, Power1/1, Power/1
  Math Function/1 -> Product/3
  Divide1/1 -> Add/2
  Constant7/1 -> Add5/1
  Add1/1 -> Math Function/1
  Add4/1 -> Divide2/2
  Gain/1 -> Add/4
  Constant3/1 -> Add3/1
  Gain1/1 -> Add2/2
  Divide3/1 -> Add1/2
  Divide2/1 -> Add1/1
  Gain2/1 -> Add4/2
  Power1/1 -> Add5/2
  Add5/1 -> Divide3/2
  Constant9/1 -> Product/1
  Product/1 -> Add6/2
  Constant8/1 -> Power1/2
  Constant1/1 -> Divide1/1
  Add2/1 -> Divide/2
  Constant2/1 -> Divide/1
  Add/1 -> Product/2
  Lambda/1 -> Gain3/1, Add2/1, Add4/1

== system RaviDFG/SM_OPALNode1/DFIG/Generator/esq---esd/F_Eds ==
  note: wb*ws
  Isq : Inport
  wg : Inport  Port=2
  Vrq : Inport  Port=3
  -1/(Trws)4 : Gain  Gain=1/(d_Tr*d_ws)
  -1/(Trws)5 : Gain  Gain=d_Kmrr
  Add3 : Sum  Inputs=-+-+
  Add5 : Sum  Inputs=-+
  Constant1 : Constant
  Integrator3 : Integrator  InitialCondition=0.48458048  UpperSaturationLimit=0.1095  LowerSaturationLimit=-0.001
  Product3 : Product  RndMeth=Zero
  wb/Ls4 : Gain  Gain=d_welb*d_ws
  wsLs4 : Gain  Gain=d_R2
  wsLs8 : Gain  Gain=1/d_ws
  Esd : Outport  VectorParamsAs1DForOutWhenUnconnected=off
  wires:
  Isq/1 -> wsLs4/1
  [esd] -> -1/(Trws)4/1
  Add3/1 -> wb/Ls4/1
  wb/Ls4/1 -> Integrator3/1
  wsLs4/1 -> Add3/1
  Product3/1 -> Add3/2
  -1/(Trws)4/1 -> Add3/3
  Vrq/1 -> -1/(Trws)5/1
  -1/(Trws)5/1 -> Add3/4
  wg/1 -> wsLs8/1
  Constant1/1 -> Add5/1
  wsLs8/1 -> Add5/2
  Add5/1 -> Product3/2
  [esq] -> Product3/1
  Integrator3/1 -> Esd/1

== system RaviDFG/SM_OPALNode1/DFIG/Generator/esq---esd/F_Eqs ==
  note: wb*ws
  Isd : Inport
  wg : Inport  Port=2
  Vrd : Inport  Port=3
  -1/(Trws)3 : Gain  Gain=d_Kmrr
  Add2 : Sum  Inputs=+-+-
  Add4 : Sum  Inputs=+-
  Constant : Constant
  Integrator2 : Integrator  InitialCondition=0.9590  UpperSaturationLimit=1  LowerSaturationLimit=-0.01
  Product2 : Product  RndMeth=Zero
  wb/Ls3 : Gain  Gain=d_welb*d_ws
  wr/ws2 : Gain  Gain=1/(d_Tr*d_ws)
  wsLs3 : Gain  Gain=d_R2
  wsLs7 : Gain  Gain=1/d_ws
  Esq : Outport  VectorParamsAs1DForOutWhenUnconnected=off
  wires:
  Isd/1 -> wsLs3/1
  [esq] -> wr/ws2/1
  Add2/1 -> wb/Ls3/1
  wb/Ls3/1 -> Integrator2/1
  Integrator2/1 -> Esq/1
  wsLs3/1 -> Add2/1
  wr/ws2/1 -> Add2/2
  Product2/1 -> Add2/3
  Vrd/1 -> -1/(Trws)3/1
  -1/(Trws)3/1 -> Add2/4
  wg/1 -> wsLs7/1
  Constant/1 -> Add4/1
  wsLs7/1 -> Add4/2
  Add4/1 -> Product2/2
  [esd] -> Product2/1

== system RaviDFG/SM_OPALNode1/DFIG/Generator/isq---isd/F_Ids ==
  Vsd : Inport
  Vrd : Inport  Port=2
  wg : Inport  Port=3
  -R2 : Gain  Gain=d_ws*d_Ls_d
  Add1 : Sum  Inputs=--+++-
  Integrator1 : Integrator  InitialCondition=d_isd  UpperSaturationLimit=1  LowerSaturationLimit=-2
  Kmrr1 : Gain  Gain=d_Kmrr
  Product1 : Product  RndMeth=Zero
  wb/Ls2 : Gain  Gain=d_welb/d_Ls_d
  wr/ws1 : Gain  Gain=1/(d_Tr*d_ws)
  wsLs2 : Gain  Gain=d_R1
  wsLs6 : Gain  Gain=1/d_ws
  Isd : Outport  VectorParamsAs1DForOutWhenUnconnected=off
  wires:
  [isq] -> -R2/1
  [isd] -> wsLs2/1
  [esq] -> wr/ws1/1
  Vrd/1 -> Kmrr1/1
  -R2/1 -> Add1/1
  wsLs2/1 -> Add1/2
  wr/ws1/1 -> Add1/3
  wsLs6/1 -> Add1/4
  Kmrr1/1 -> Add1/5
  Add1/1 -> wb/Ls2/1
  Product1/1 -> wsLs6/1
  wg/1 -> Product1/2
  [esd] -> Product1/1
  Vsd/1 -> Add1/6
  wb/Ls2/1 -> Integrator1/1
  Integrator1/1 -> Isd/1

== system RaviDFG/SM_OPALNode1/DFIG/Generator/isq---isd/F_Iqs ==
  Vsq : Inport
  Vrq : Inport  Port=2
  wg : Inport  Port=3
  1/(Trws) : Gain  Gain=1/(d_Tr*d_ws)
  Add : Sum  Inputs=-++--+
  Integrator : Integrator  InitialCondition=d_isq  UpperSaturationLimit=1  LowerSaturationLimit=-0.1
  Kmrr : Gain  Gain=d_Kmrr
  Product : Product  RndMeth=Zero
  R1 : Gain  Gain=d_R1
  wb/Ls1 : Gain  Gain=d_welb/d_Ls_d
  wsLs1 : Gain  Gain=d_ws*d_Ls_d
  wsLs5 : Gain  Gain=1/d_ws
  Isq : Outport  VectorParamsAs1DForOutWhenUnconnected=off
  wires:
  [isq] -> R1/1
  [isd] -> wsLs1/1
  [esd] -> 1/(Trws)/1
  Vrq/1 -> Kmrr/1
  R1/1 -> Add/1
  wsLs1/1 -> Add/2
  Product/1 -> wsLs5/1
  1/(Trws)/1 -> Add/4
  Vsq/1 -> Add/5
  Kmrr/1 -> Add/6
  Add/1 -> wb/Ls1/1
  wb/Ls1/1 -> Integrator/1
  Integrator/1 -> Isq/1
  [esq] -> Product/1
  wg/1 -> Product/2
  wsLs5/1 -> Add/3
